simulink model "flightControlSystem"  (R2021b)
settings: Solver=ode3  StartTime=0  StopTime=TFinal  FixedStep=Ts  RelTol=1e-3  EnableMultiTasking=on
undefined symbols (not defined in the file): codertarget, Controller, DiscIntNeverNeededParam, Discrete, Estimator, g, init, Sensors, Time, Ts, var_acc_angle_N, var_bias_gyr_N, var_gyro_p_N, Vehicle
libraries: simulink x44, slpidlib x4, ctrlSharedLib x4, sharedtransform x3, rllib x1, fuzblock x1, simulink_need_slupdate x1, parrotlib x1
(part 3 of 3)

== system flightControlSystem/Flight Control System/Controller/Altitude Controller/reward/Subsystem2/Subsystem1/-1 < e ==
  Action Port : Inport
  <dz> : Inport  Port=2
  -500 : Subsystem  TreatAsAtomicUnit=on
  500 : Subsystem  TreatAsAtomicUnit=on
  Constant : Constant
  If Action Subsystem1 : Subsystem  TreatAsAtomicUnit=on
  If1 : If  IfExpression=u1 < 0
  Sum2 : Sum  Inputs=|++
  Out1 : Outport
  wires:
  <dz>/1 -> If Action Subsystem1/1(In1)
  -500/1(Out1) -> Sum2/2
  Action Port/1 -> If Action Subsystem1/Action
  If Action Subsystem1/1(Out1) -> If1/1
  500/1(Out1) -> Sum2/1
  If1/2 -> -500/Action
  If1/1 -> 500/Action
  Constant/1 -> -500/1(In1), 500/1(In1)
  Sum2/1 -> Out1/1

== system flightControlSystem/Flight Control System/Controller/Altitude Controller/reward/Subsystem2/Subsystem1/If Action Subsystem1 ==
  In1 : Inport
  Action Port : ActionPort  ActionPortLabel=else
  Gain8 : Gain  Gain=1000
  Out1 : Outport
  wires:
  In1/1 -> Gain8/1
  Gain8/1 -> Out1/1

== system flightControlSystem/Flight Control System/Controller/Altitude Controller/reward/Subsystem2/Subsystem1/If Action Subsystem3 ==
  In1 : Inport
  Action Port : ActionPort  ActionPortLabel=else
  Out1 : Outport
  wires:
  In1/1 -> Out1/1

== system flightControlSystem/Flight Control System/Controller/Altitude Controller/reward/Subsystem2/Subsystem1/e < -1 ==
  Action Port : Inport
  <dz> : Inport  Port=2
  e : Inport  Port=3
  -I : Subsystem  TreatAsAtomicUnit=on
  100 : Subsystem  TreatAsAtomicUnit=on
  Constant : Constant
  I : Subsystem
  If Action Subsystem1 : Subsystem  TreatAsAtomicUnit=on
  If1 : If  IfExpression=u1 < 0
  Sum2 : Sum  Inputs=|++
  Out1 : Outport
  wires:
  <dz>/1 -> If Action Subsystem1/1(In1)
  -I/1(Out1) -> Sum2/2
  Action Port/1 -> If Action Subsystem1/Action
  If Action Subsystem1/1(Out1) -> If1/1
  100/1(Out1) -> Sum2/1
  If1/2 -> -I/Action
  If1/1 -> 100/Action
  Constant/1 -> 100/1(In1)
  Sum2/1 -> Out1/1
  e/1 -> I/1(In1)
  I/1(IAE1) -> -I/1(In1)  "I"

== system flightControlSystem/Flight Control System/Controller/Altitude Controller/reward/Subsystem2/Subsystem1/e > 1 ==
  Action Port : Inport
  <dz> : Inport  Port=2
  e : Inport  Port=3
  -I : Subsystem  TreatAsAtomicUnit=on
  100 : Subsystem  TreatAsAtomicUnit=on
  Constant : Constant
  I : Subsystem
  If Action Subsystem1 : Subsystem  TreatAsAtomicUnit=on
  If1 : If  IfExpression=u1 < 0
  Sum2 : Sum  Inputs=|++
  Out1 : Outport
  wires:
  <dz>/1 -> If Action Subsystem1/1(In1)
  100/1(Out1) -> Sum2/2
  Action Port/1 -> If Action Subsystem1/Action
  If Action Subsystem1/1(Out1) -> If1/1
  -I/1(Out1) -> Sum2/1
  If1/2 -> 100/Action
  If1/1 -> -I/Action
  Constant/1 -> 100/1(In1)
  Sum2/1 -> Out1/1
  e/1 -> I/1(e)
  I/1(IAE1) -> -I/1(IAE1)  "I"

== system flightControlSystem/Flight Control System/Controller/Altitude Controller/reward/Subsystem2/Subsystem1/ 1 > e/-500 ==
  In1 : Inport
  Action Port : ActionPort  ActionPortLabel=else
  Gain : Gain  Gain=-500
  Out1 : Outport
  wires:
  In1/1 -> Gain/1
  Gain/1 -> Out1/1

== system flightControlSystem/Flight Control System/Controller/Altitude Controller/reward/Subsystem2/Subsystem1/ 1 > e/500 ==
  In1 : Inport
  Action Port : ActionPort  ActionPortLabel="if(u1 >  0)"
  Gain : Gain  Gain=500
  Out1 : Outport
  wires:
  In1/1 -> Gain/1
  Gain/1 -> Out1/1

== system flightControlSystem/Flight Control System/Controller/Altitude Controller/reward/Subsystem2/Subsystem1/ 1 > e/If Action Subsystem1 ==
  In1 : Inport
  Action Port : ActionPort  ActionPortLabel=elseif(1 >= u1 > 0.1)
  Out1 : Outport
  wires:
  In1/1 -> Out1/1

== system flightControlSystem/Flight Control System/Controller/Altitude Controller/reward/Subsystem2/Subsystem1/-1 < e/-500 ==
  In1 : Inport
  Action Port : ActionPort  ActionPortLabel=else
  Gain : Gain  Gain=-500
  Out1 : Outport
  wires:
  In1/1 -> Gain/1
  Gain/1 -> Out1/1

== system flightControlSystem/Flight Control System/Controller/Altitude Controller/reward/Subsystem2/Subsystem1/-1 < e/500 ==
  In1 : Inport
  Action Port : ActionPort  ActionPortLabel=if(u1 < 0)
  Gain : Gain  Gain=500
  Out1 : Outport
  wires:
  In1/1 -> Gain/1
  Gain/1 -> Out1/1

== system flightControlSystem/Flight Control System/Controller/Altitude Controller/reward/Subsystem2/Subsystem1/-1 < e/If Action Subsystem1 ==
  In1 : Inport
  Action Port : ActionPort  ActionPortLabel=if(-1 <= u1 < -0.1)
  Out1 : Outport
  wires:
  In1/1 -> Out1/1

== system flightControlSystem/Flight Control System/Controller/Altitude Controller/reward/Subsystem2/Subsystem1/e < -1/-I ==
  In1 : Inport
  Action Port : ActionPort  ActionPortLabel=else
  Gain : Gain  Gain=-1
  Out1 : Outport
  wires:
  In1/1 -> Gain/1
  Gain/1 -> Out1/1

== system flightControlSystem/Flight Control System/Controller/Altitude Controller/reward/Subsystem2/Subsystem1/e < -1/100 ==
  In1 : Inport
  Action Port : ActionPort  ActionPortLabel=if(u1 < 0)
  Gain : Gain  Gain=100
  Out1 : Outport
  wires:
  In1/1 -> Gain/1
  Gain/1 -> Out1/1

== system flightControlSystem/Flight Control System/Controller/Altitude Controller/reward/Subsystem2/Subsystem1/e < -1/I ==
  In1 : Inport
  IAE : Subsystem
      mask help:
      | IAE performacne index
      |
      | output = int |input| dt
      mask Display:
      | disp('IAE')
      | port_label('input',1,'e')
      | port_label('output',1,'iae')
  ISE : Subsystem
      mask help:
      | ISE performance index
      |
      | output = int (input)^2 dt
      mask Display:
      | disp('ISE')
      | port_label('input',1,'e')
      | port_label('output',1,'ise')
  ITAE : Subsystem  Commented=on
      mask help:
      | ITAE performance index
      |
      | output = int t|input| dt
      mask Display:
      | disp('ITAE')
      | port_label('input',1,'e')
      | port_label('output',1,'itae')
  Sum1 : Sum  Inputs=+++
  IAE1 : Outport
  wires:
  ITAE/1(Out1) -> Sum1/1
  In1/1 -> IAE/1(In1), ITAE/1(In1), ISE/1(In1)
  Sum1/1 -> IAE1/1  "IAE"
  IAE/1(Out1) -> Sum1/2
  ISE/1(Out1) -> Sum1/3

== system flightControlSystem/Flight Control System/Controller/Altitude Controller/reward/Subsystem2/Subsystem1/e < -1/If Action Subsystem1 ==
  In1 : Inport
  Action Port : ActionPort  ActionPortLabel=if(u1 < -1)
  Out1 : Outport
  wires:
  In1/1 -> Out1/1

== system flightControlSystem/Flight Control System/Controller/Altitude Controller/reward/Subsystem2/Subsystem1/e > 1/-I ==
  IAE1 : Inport
  Action Port : ActionPort  ActionPortLabel=if(u1 < 0)
  Gain : Gain  Gain=-1
  Out1 : Outport
  wires:
  IAE1/1 -> Gain/1
  Gain/1 -> Out1/1

== system flightControlSystem/Flight Control System/Controller/Altitude Controller/reward/Subsystem2/Subsystem1/e > 1/100 ==
  In1 : Inport
  Action Port : ActionPort  ActionPortLabel=else
  Gain : Gain  Gain=100
  Out1 : Outport
  wires:
  In1/1 -> Gain/1
  Gain/1 -> Out1/1

== system flightControlSystem/Flight Control System/Controller/Altitude Controller/reward/Subsystem2/Subsystem1/e > 1/I ==
  e : Inport
  IAE : Subsystem
      mask help:
      | IAE performacne index
      |
      | output = int |input| dt
      mask Display:
      | disp('IAE')
      | port_label('input',1,'e')
      | port_label('output',1,'iae')
  ISE : Subsystem
      mask help:
      | ISE performance index
      |
      | output = int (input)^2 dt
      mask Display:
      | disp('ISE')
      | port_label('input',1,'e')
      | port_label('output',1,'ise')
  ITAE : Subsystem  Commented=on
      mask help:
      | ITAE performance index
      |
      | output = int t|input| dt
      mask Display:
      | disp('ITAE')
      | port_label('input',1,'e')
      | port_label('output',1,'itae')
  Sum1 : Sum  Inputs=+++
  IAE1 : Outport
  wires:
  ITAE/1(Out1) -> Sum1/1
  e/1 -> IAE/1(In1), ITAE/1(In1), ISE/1(In1)
  Sum1/1 -> IAE1/1  "IAE"
  IAE/1(Out1) -> Sum1/2
  ISE/1(Out1) -> Sum1/3

== system flightControlSystem/Flight Control System/Controller/Altitude Controller/reward/Subsystem2/Subsystem1/e > 1/If Action Subsystem1 ==
  In1 : Inport
  Action Port : ActionPort  ActionPortLabel=elseif(u1 > 1)
  Out1 : Outport
  wires:
  In1/1 -> Out1/1

== system flightControlSystem/Flight Control System/Controller/Altitude Controller/reward/Subsystem2/Subsystem1/e < -1/I/IAE ==
  In1 : Inport
  Abs : Abs
  Discrete-Time Integrator : DiscreteIntegrator  SampleTime=-1  ICPrevOutput=DiscIntNeverNeededParam  ICPrevScaledInput=DiscIntNeverNeededParam
  Integrator : Integrator  Commented=on
  Out1 : Outport
  wires:
  In1/1 -> Abs/1
  Abs/1 -> Discrete-Time Integrator/1
  Discrete-Time Integrator/1 -> Out1/1

== system flightControlSystem/Flight Control System/Controller/Altitude Controller/reward/Subsystem2/Subsystem1/e < -1/I/ISE ==
  In1 : Inport
  Discrete-Time Integrator : DiscreteIntegrator  SampleTime=-1  ICPrevOutput=DiscIntNeverNeededParam  ICPrevScaledInput=DiscIntNeverNeededParam
  Integrator : Integrator  Commented=on
  Math Function : Math  Operator=square  SignedPower=on  SaturateOnIntegerOverflow=on
  Out1 : Outport
  wires:
  In1/1 -> Math Function/1
  Math Function/1 -> Discrete-Time Integrator/1
  Discrete-Time Integrator/1 -> Out1/1

== system flightControlSystem/Flight Control System/Controller/Altitude Controller/reward/Subsystem2/Subsystem1/e < -1/I/ITAE ==
  In1 : Inport
  Abs : Abs
  Clock : Clock
      settings: Decimation=100
  Discrete-Time Integrator : DiscreteIntegrator  SampleTime=-1  ICPrevOutput=DiscIntNeverNeededParam  ICPrevScaledInput=DiscIntNeverNeededParam
  Divide : Product  Inputs=**
  Integrator : Integrator  Commented=on
  Out1 : Outport
  wires:
  In1/1 -> Abs/1
  Divide/1 -> Discrete-Time Integrator/1
  Abs/1 -> Divide/1
  Clock/1 -> Divide/2
  Discrete-Time Integrator/1 -> Out1/1

== system flightControlSystem/Flight Control System/Controller/Altitude Controller/reward/Subsystem2/Subsystem1/e > 1/I/IAE ==
  In1 : Inport
  Abs : Abs
  Discrete-Time Integrator : DiscreteIntegrator  SampleTime=-1  ICPrevOutput=DiscIntNeverNeededParam  ICPrevScaledInput=DiscIntNeverNeededParam
  Integrator : Integrator  Commented=on
  Out1 : Outport
  wires:
  In1/1 -> Abs/1
  Abs/1 -> Discrete-Time Integrator/1
  Discrete-Time Integrator/1 -> Out1/1

== system flightControlSystem/Flight Control System/Controller/Altitude Controller/reward/Subsystem2/Subsystem1/e > 1/I/ISE ==
  In1 : Inport
  Discrete-Time Integrator : DiscreteIntegrator  SampleTime=-1  ICPrevOutput=DiscIntNeverNeededParam  ICPrevScaledInput=DiscIntNeverNeededParam
  Integrator : Integrator  Commented=on
  Math Function : Math  Operator=square  SignedPower=on  SaturateOnIntegerOverflow=on
  Out1 : Outport
  wires:
  In1/1 -> Math Function/1
  Math Function/1 -> Discrete-Time Integrator/1
  Discrete-Time Integrator/1 -> Out1/1

== system flightControlSystem/Flight Control System/Controller/Altitude Controller/reward/Subsystem2/Subsystem1/e > 1/I/ITAE ==
  In1 : Inport
  Abs : Abs
  Clock : Clock
      settings: Decimation=100
  Discrete-Time Integrator : DiscreteIntegrator  SampleTime=-1  ICPrevOutput=DiscIntNeverNeededParam  ICPrevScaledInput=DiscIntNeverNeededParam
  Divide : Product  Inputs=**
  Integrator : Integrator  Commented=on
  Out1 : Outport
  wires:
  In1/1 -> Abs/1
  Divide/1 -> Discrete-Time Integrator/1
  Abs/1 -> Divide/1
  Clock/1 -> Divide/2
  Discrete-Time Integrator/1 -> Out1/1

== matlab function flightControlSystem/Flight Control System/Controller/Position Controller/Position error transformation (Earth to Body frame) ==
  data: yaw input; xy_err_earth input; xy_err_body output
function xy_err_body = fcn(yaw,xy_err_earth)

transformation = [cos(yaw), sin(yaw); -sin(yaw),  cos(yaw)];
xy_err_body = transformation * xy_err_earth;


end
